simulink library "dspmlti4"  (Simulink 8.2)
settings: Solver=ode45  SolverMode=SingleTasking  StartTime=0.0  StopTime=10.0  RelTol=1e-3
undefined symbols (not defined in the file): Hm_decim, Hm_firdecim, Hm_firinterp, Hm_firsrc, Hm_interp
libraries: simulink x1
settings Model: RequirementInfo=9  Creator=tbryan  LastModifiedBy=jibrahim  CovMetricSettings=d  ExtModeAutoUpdateStatusClock=off

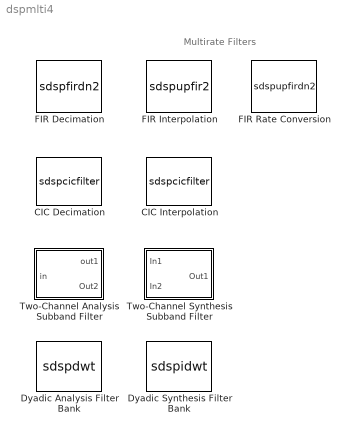
== system dspmlti4 ==
  note: Multirate Filters
  CIC Decimation : S-Function  DialogController=dspdialog.CICDecimation  FunctionName=sdspcicfilter  Parameters=filtFrom,a.ftype,a.R,a.M,a.N,filterInternals,a.section2NWL,a.section2NFL,a.outWL,a.outFL,a.states,framing,1,RateOptions,a.InputWL,a.InputFL  EnableBusSupport=off  mask(CIC Decimation){filtFrom=Dialog, filtobj=Hm_decim, ftype=Decimator, R=2, M=1, N=2, filterInternals=Full precision, BPS=[16 16 16 16], FLPS=0, outputWordLength=32, outputFracLength=0, launchFVT=off, framing=Maintain input frame rate, RateOptions=Enforce single-rate}
      mask prompts: filtFrom "Filter specified via:"; filtobj "Multirate filter variable:"; ftype "Filter structure:"; R "Decimation factor (R):"; M "Differential delay (M):"; N "Number of stages (N):"; filterInternals "Filter internals:"; BPS "Word length for each of the (2*N) filter sections:"; FLPS "Fraction length for each of the (2*N) filter sections:"; outputWordLength "Output word length:"; outputFracLength "Output fraction length:"; launchFVT "Launch Filter Visualization Tool (FVTool)"; RateOptions "Rate options:"
      mask help:
      | Apply a Cascaded Integrator-Comb Decimator filter to the input signal.
      |
      | The inputs and outputs of this block have a signed fixed-point data type with zero bias. You must have a Fixed-Point Designer license to use this block.
      mask init:
      | if filtFrom == 1
      |   str  = dspblkcicfilter('icon',gcbh,filtFrom,'Decimation');
      |   a = dspblkcicfilter('init',gcbh,filtFrom,R,M,N,BPS,FLPS,outputWordLength,outputFracLength,filterInternals);
      | else
      |   str  = dspblkcicfilter('icon',gcbh,filtFrom);
      |   a = dspblkcicfilter('init',gcbh,filtFrom,'Decimation',filtobj);
      | end
      | dspblkcicfilter('initCICDecim',gcbh,filtFrom);
      settings: DeleteFcn=dspLinkFVTool2Mask(gcbh,'close')
      mask Help: eval('blocksethelp');
      mask TypeOptions filtFrom: Dialog | Multirate object in workspace
      mask TypeOptions ftype: Decimator | Zero-latency decimator
      mask TypeOptions filterInternals: Full precision | Minimum section word lengths | Specify word lengths | Binary point scaling
      mask TypeOptions framing: Maintain input frame rate | Maintain input frame size
      mask TypeOptions RateOptions: Enforce single-rate processing | Allow multirate processing | Inherit from input (this choice will be removed - see release notes)
      mask Display: disp(str);
  CIC Interpolation : S-Function  DialogController=dspdialog.CICInterpolation  FunctionName=sdspcicfilter  Parameters=filtFrom,a.ftype,a.R,a.M,a.N,filterInternals,a.section2NWL,a.section2NFL,a.outWL,a.outFL,a.states,framing,InputProcessing,1,a.InputWL, a.InputFL  EnableBusSupport=off  mask(CIC Interpolation){filtFrom=Dialog, filtobj=Hm_interp, ftype=Interpolator, R=2, M=1, N=2, filterInternals=Full precision, BPS=[16 16 16 16], FLPS=0, outputWordLength=32, outputFracLength=0, launchFVT=off, framing=Enforce single-rate, InputProcessing=Columns as channels (frame based)}
      mask prompts: filtFrom "Filter specified via:"; filtobj "Multirate filter variable:"; ftype "Filter structure:"; R "Interpolation factor (R):"; M "Differential delay (M):"; N "Number of stages (N):"; filterInternals "Filter internals:"; BPS "Word length for each of the (2*N) filter stages:"; FLPS "Fraction length for each of the (2*N) filter stages:"; outputWordLength "Output word length:"; outputFracLength "Output fraction length:"; launchFVT "Launch Filter Visualization Tool (FVTool)"; InputProcessing "Input processing:"
      mask help:
      | Apply a Cascaded Integrator-Comb Interpolator filter to the input signal.
      |
      | The inputs and outputs of this block have a signed fixed-point data type with zero bias. You must have a Fixed-Point Designer license to use this block.
      mask init:
      | if filtFrom == 1
      |   str  = dspblkcicfilter('icon',gcbh,filtFrom,'Interpolation');
      |   a = dspblkcicfilter('init',gcbh,filtFrom,R,M,N,BPS,FLPS,outputWordLength,outputFracLength,filterInternals);
      | else
      |   str  = dspblkcicfilter('icon',gcbh,filtFrom);
      |   a = dspblkcicfilter('init',gcbh,filtFrom,'Interpolation',filtobj);
      | end
      | framing = dspblkcicfilter('initCICInterp',gcbh,filtFrom,framing);
      settings: DeleteFcn=dspLinkFVTool2Mask(gcbh,'close')
      mask Help: eval('blocksethelp');
      mask TypeOptions filtFrom: Dialog | Multirate object in workspace
      mask TypeOptions ftype: Interpolator | Zero-latency interpolator
      mask TypeOptions filterInternals: Full precision | Minimum section word lengths | Specify word lengths | Binary point scaling
      mask TypeOptions framing: Enforce single-rate processing | Allow multirate processing | Maintain input frame rate | Maintain input frame size
      mask TypeOptions InputProcessing: Columns as channels (frame based) | Elements as channels (sample based) | Inherited (this choice will be removed - see release notes)
      mask Display: disp(str);
  Dyadic Analysis Filter Bank : S-Function  FunctionName=sdspdwt  Parameters=phl, phh, NumLevels, tree, Output  EnableBusSupport=off  mask(Dyadic Analysis Filter Bank){Wname=User-defined, OrdRec_ordDec=[1 / 1], Order=2, LPF=[0.0352   -0.0854   -0.1350   0.4599   0.8069   0.3327], HPF=[-0.3327    0.8069   -0.4599   -0.1350    0.0854    0.0352], NumLevels=2, tree=Asymmetric, Output=Multiple ports}
      mask prompts: Wname "Filter:"; OrdRec_ordDec "Filter order [synthesis / analysis]:"; Order "Wavelet order:"; LPF "Lowpass FIR filter coefficients:"; HPF "Highpass FIR filter coefficients:"; NumLevels "Number of levels:"; tree "Tree structure:"
      mask help:
      | Compute the Discrete Wavelet Transform or decompose a signal into subbands with smaller bandwidths and slower sample rates. This block uses a filter bank with lowpass and highpass FIR filters that you specify either directly on the block mask, or using wavelets from the Wavelet Toolbox. The lowpass and highpass filters are usually half-band filters designed to complement each other.
      |
      | Inputs are always interpreted as frames. The frame size must be a multiple of 2^n, where you specify n in the 'Number of levels' parameter. When the 'Output' parameter is set to 'Multiple ports', the block outputs each subband from a different port as a vector or matrix. The topmost port outputs the subband with the highest frequency band. When the 'Output' parameter is set to 'Single port', the block outputs one vector or matrix of concatenated subbands.
      mask init:
      | [x,y, str] = dspblkdwt('icon');
      | wname_str = get_param(gcb, 'Wname');
      | OrdRec_ordDec_str = get_param(gcb, 'OrdRec_ordDec');
      | [phl, phh] = dspblkdwt('init', true, LPF, HPF, tree, wname_str, Order, OrdRec_ordDec_str);
      mask Help: eval('blocksethelp');
      mask TypeOptions Wname: User-defined | Haar | Daubechies | Symlets | Coiflets | Biorthogonal | Reverse Biorthogonal | Discrete Meyer
      mask Callback Wname: dspblkdwt
      mask TypeOptions OrdRec_ordDec: [1 / 1] | [1 / 3] | [1 / 5] | [2 / 2] | [2 / 4] | [2 / 6] | [2 / 8] | [3 / 1] | [3 / 3] | [3 / 5] | [3 / 7] | [3 / 9] | [4 / 4] | [5 / 5] | [6 / 8]
      mask TypeOptions tree: Asymmetric | Symmetric
      mask TypeOptions Output: Single port | Multiple ports
      mask Display:
      | plot(x,y)
      | text(0.08,0.1,str)
  Dyadic Synthesis Filter Bank : S-Function  FunctionName=sdspidwt  Parameters=phl, phh, NumLevels, tree, Input  EnableBusSupport=off  mask(Dyadic Synthesis Filter Bank){Wname=User-defined, OrdRec_ordDec=[1 / 1], Order=2, LPF=[0.3327    0.8069    0.4599   -0.1350   -0.0854    0.0352], HPF=[0.0352    0.0854   -0.1350   -0.4599    0.8069   -0.3327], NumLevels=2, tree=Asymmetric, Input=Multiple ports}
      mask prompts: Wname "Filter:"; OrdRec_ordDec "Filter order [synthesis, analysis]:"; Order "Wavelet order:"; LPF "Lowpass FIR filter coefficients:"; HPF "Highpass FIR filter coefficients:"; NumLevels "Number of levels:"; tree "Tree Structure:"
      mask help:
      | Compute the Inverse Discrete Wavelet Transform or reconstruct a signal from subbands with smaller bandwidths and slower sample rates. This block uses a filter bank with lowpass and highpass FIR filters that you specify either directly on the block mask, or using wavelets from the Wavelet Toolbox. The lowpass and highpass filters are usually half-band filters designed to complement each other.
      |
      | When 'Input' is set to 'Multiple ports', you must provide each subband to the block through a different input port as a vector or matrix. You should input the highest frequency band through the topmost port. When 'Input' is set to 'Single port', the block input must be a vector or matrix of concatenated subbands.
      mask init:
      | [x,y,str] = dspblkidwt('icon');
      | wname_str = get_param(gcb, 'Wname');
      | OrdRec_ordDec_str = get_param(gcb, 'OrdRec_ordDec');
      | [phl, phh] = dspblkidwt('init', true, LPF, HPF, tree, wname_str, Order, OrdRec_ordDec_str);
      mask Help: eval('blocksethelp');
      mask TypeOptions Wname: User-defined | Haar | Daubechies | Symlets | Coiflets | Biorthogonal | Reverse Biorthogonal | Discrete Meyer
      mask Callback Wname: dspblkidwt
      mask TypeOptions OrdRec_ordDec: [1 / 1] | [1 / 3] | [1 / 5] | [2 / 2] | [2 / 4] | [2 / 6] | [2 / 8] | [3 / 1] | [3 / 3] | [3 / 5] | [3 / 7] | [3 / 9] | [4 / 4] | [5 / 5] | [6 / 8]
      mask TypeOptions tree: Asymmetric | Symmetric
      mask TypeOptions Input: Single port | Multiple ports
      mask Display:
      | plot(x,y)
      | text(0.08,0.1,str)
  FIR Decimation : S-Function  DialogController=dspdialog.FIRDecimation  DialogControllerArgs=DataTag3  FunctionName=sdspfirdn2  Parameters=a.CoeffSource,a.h,a.D,framing,InputProcessing,inputOffset,a.outBufIC,a.filtStruct,dtInfo.arithmetic,dtInfo.inputWordLength,dtInfo.inputFracLength,firstCoeffMin,firstCoeffMax,outputMin,outputMax,dtInfo.firstCoeffMode,dtInfo.firstCoeffWordLength,dtInfo.firstCoeffFracLength,dtInfo.prodOutputMode,dtInfo.prodOutputWordLength,dtInfo.prodOutputFracLength,dtInfo.accumMode,dtInfo.accumWordLength,dtInfo.accumFracLength,dtInfo.outputMode,dtInfo.outputWordLength,dtInfo.outputFracLength,dtInfo.roundingMode,dtInfo.overflowMode  EnableBusSupport=off  mask(FIR Decimation){h=fir1(35,0.4), D=2, filtStruct=Direct form, framing=Enforce single-rate, inputOffset=0, outputBufInitCond=0, InputProcessing=Columns as channels (frame based), additionalParams=off, allowOverrides=off, firstCoeffMode=Same word length as input, firstCoeffWordLength=16, firstCoeffFracLength=15, firstCoeffDataTypeStr=Inherit: Same word length as input, firstCoeffLastDataTypeStr=Inherit: Same word length as input, firstCoeffMin=[], firstCoeffMax=[], outputMode=Same as accumulator, outputWordLength=16, outputFracLength=15, outputDataTypeStr=Inherit: Same as accumulator, outputLastDataTypeStr=Inherit: Same as accumulator, outputMin=[], outputMax=[], accumMode=Inherit via internal rule, accumWordLength=32, accumFracLength=30, accumDataTypeStr=Inherit: Inherit via internal rule, accumLastDataTypeStr=Inherit: Inherit via internal rule, prodOutputMode=Inherit via internal rule, prodOutputWordLength=32, prodOutputFracLength=30, prodOutputDataTypeStr=Inherit: Inherit via internal rule, prodOutputLastDataTypeStr=Inherit: Inherit via internal rule, roundingMode=Floor, overflowMode=off, LockScale=off, FilterSource=Specify via dialog, FilterObject=Hm_firdecim}
      mask prompts: h "FIR filter coefficients:"; D "Decimation factor:"; filtStruct "Filter structure:"; inputOffset "Input offset:"; outputBufInitCond "Output buffer initial conditions:"; InputProcessing "Input processing:"; additionalParams "--------------- Show additional parameters ---------------"; allowOverrides "Allow overrides from DSP Fixed-Point Attributes blocks"; firstCoeffMode "Fixed-point coefficient attributes:"; firstCoeffWordLength "Coefficient word length:"; firstCoeffFracLength "Coefficient fraction length:"; firstCoeffDataTypeStr "Coefficients data type string:"; firstCoeffLastDataTypeStr "Last coefficients data type string:"; firstCoeffMin "Coefficients minimum:"; firstCoeffMax "Coefficients maximum:"; outputMode "Fixed-point output attributes:"; outputWordLength "Output word length:"; outputFracLength "Output fractional length:"; outputDataTypeStr "Output data type string:"; outputLastDataTypeStr "Last output data type string:"; outputMin "Output minimum:"; outputMax "Output maximum:"; accumMode "Fixed-point accumulator attributes:"; accumWordLength "Accumulator word length:"; accumFracLength "Accumulator fraction length:"; accumDataTypeStr "Accum data type string:"; accumLastDataTypeStr "Last accum data type string:"; prodOutputMode "Fixed-point product output attributes:"; prodOutputWordLength "Product output word length:"; prodOutputFracLength "Product output fraction length:"; prodOutputDataTypeStr "ProdOutput data type string:"; prodOutputLastDataTypeStr "Last prodOutput data type string:"; roundingMode "Round integer calculations towards:"; overflowMode "Saturate on integer overflow"; LockScale "Lock scaling"; FilterSource "Coefficient source:"; FilterObject "Filter object:"
      mask help: Apply an FIR filter to the input signal, then downsample the signal by an integer-valued factor. The block implements the FIR filter using a polyphase filter structure.
      mask init:
      | dtRows = dspblkGetFIRMultirateFiltersDTRowInfo();
      | if FilterSource == 1
      |     str = dspblkfirdn2(gcbh,'icon',FilterSource,D);
      |     [a,dtInfo,framing] = dspblkfirdn2(gcbh,'setup',FilterSource,dtRows,h,D,filtStruct,outputBufInitCond,framing);
      | else
      |     str = dspblkfirdn2(gcbh,'icon',FilterSource,FilterObject);
      |     [a,dtInfo,framing] = dspblkfirdn2(gcbh,'setup',FilterSource,FilterObject,framing);
      | end
      | dspblkfirdn2(gcbh,'init',FilterSource);
      settings: DeleteFcn=dspLinkFVTool2Mask(gcbh,'close')
      mask Help: eval('blocksethelp');
      mask TypeOptions filtStruct: Direct form | Direct form transposed
      mask TypeOptions framing: Enforce single-rate processing | Allow multirate processing | Maintain input frame size | Maintain input frame rate
      mask TypeOptions InputProcessing: Columns as channels (frame based) | Elements as channels (sample based) | Inherited (this choice will be removed - see release notes)
      mask TypeOptions firstCoeffMode: Same word length as input | Specify word length | Binary point scaling | Slope and bias scaling | User-defined
      mask TypeOptions outputMode: Same as accumulator | Same as product output | Same as input | Binary point scaling | Slope and bias scaling | User-defined
      mask TypeOptions accumMode: Inherit via internal rule | Same as product output | Same as input | Binary point scaling | Slope and bias scaling | User-defined
      mask TypeOptions prodOutputMode: Inherit via internal rule | Same as input | Binary point scaling | Slope and bias scaling | User-defined
      mask TypeOptions roundingMode: Ceiling | Convergent | Floor | Nearest | Round | Simplest | Zero
      mask TypeOptions FilterSource: Specify via dialog | Filter object
      mask Display: disp(str)
  FIR Interpolation : S-Function  DialogController=dspdialog.FIRInterpolation  DialogControllerArgs=DataTag5  FunctionName=sdspupfir2  Parameters=a.CoeffSource,a.h,a.L,framing,InputProcessing,a.outBufIC,dtInfo.arithmetic,dtInfo.inputWordLength,dtInfo.inputFracLength,firstCoeffMin,firstCoeffMax,outputMin,outputMax,dtInfo.firstCoeffMode,dtInfo.firstCoeffWordLength,dtInfo.firstCoeffFracLength,dtInfo.prodOutputMode,dtInfo.prodOutputWordLength,dtInfo.prodOutputFracLength,dtInfo.accumMode,dtInfo.accumWordLength,dtInfo.accumFracLength,dtInfo.outputMode,dtInfo.outputWordLength,dtInfo.outputFracLength,dtInfo.roundingMode,dtInfo.overflowMode  EnableBusSupport=off  mask(FIR Interpolation){h=fir1(15,1/4), L=3, framing=Enforce single-rate processing, outputBufInitCond=0, InputProcessing=Columns as channels (frame based), additionalParams=off, allowOverrides=on, firstCoeffMode=Same word length as input, firstCoeffWordLength=16, firstCoeffFracLength=15, firstCoeffDataTypeStr=Inherit: Same word length as input, firstCoeffLastDataTypeStr=Inherit: Same word length as input, firstCoeffMin=[], firstCoeffMax=[], outputMode=Same as accumulator, outputWordLength=16, outputFracLength=15, outputDataTypeStr=Inherit: Same as accumulator, outputLastDataTypeStr=Inherit: Same as accumulator, outputMin=[], outputMax=[], accumMode=Inherit via internal rule, accumWordLength=32, accumFracLength=30, accumDataTypeStr=Inherit: Inherit via internal rule, accumLastDataTypeStr=Inherit: Inherit via internal rule, prodOutputMode=Inherit via internal rule, prodOutputWordLength=32, prodOutputFracLength=30, prodOutputDataTypeStr=Inherit: Inherit via internal rule, prodOutputLastDataTypeStr=Inherit: Inherit via internal rule, roundingMode=Floor, overflowMode=off, LockScale=off, FilterSource=Specify via dialog, FilterObject=Hm_firinterp}
      mask prompts: h "FIR filter coefficients:"; L "Interpolation factor:"; outputBufInitCond "Output buffer initial conditions:"; InputProcessing "Input processing:"; additionalParams "--------------- Show additional parameters ---------------"; allowOverrides "Allow overrides from DSP Fixed-Point Attributes blocks"; firstCoeffMode "Fixed-point coefficient attributes:"; firstCoeffWordLength "Coefficient word length:"; firstCoeffFracLength "Coefficient fraction length:"; firstCoeffDataTypeStr "Coefficients data type string:"; firstCoeffLastDataTypeStr "Last coefficients data type string:"; firstCoeffMin "Coefficients minimum:"; firstCoeffMax "Coefficients maximum:"; outputMode "Fixed-point output attributes:"; outputWordLength "Output word length:"; outputFracLength "Output fractional length:"; outputDataTypeStr "Output data type string:"; outputLastDataTypeStr "Last output data type string:"; outputMin "Output minimum:"; outputMax "Output maximum:"; accumMode "Fixed-point accumulator attributes:"; accumWordLength "Accumulator word length:"; accumFracLength "Accumulator fraction length:"; accumDataTypeStr "Accum data type string:"; accumLastDataTypeStr "Last accum data type string:"; prodOutputMode "Fixed-point product output attributes:"; prodOutputWordLength "Product output word length:"; prodOutputFracLength "Product output fraction length:"; prodOutputDataTypeStr "ProdOutput data type string:"; prodOutputLastDataTypeStr "Last prodOutput data type string:"; roundingMode "Round integer calculations towards:"; overflowMode "Saturate on integer overflow"; LockScale "Lock scaling"; FilterSource "Coefficient source:"; FilterObject "Filter object:"
      mask help: Upsample the input signal by an integer-valued factor, then apply an FIR filter. The block scales the filter coefficients by the interpolation factor and implements the FIR filter using a polyphase structure.
      mask init:
      | dtRows = dspblkGetFIRMultirateFiltersDTRowInfo();
      | if FilterSource == 1
      |     str = dspblkupfir2(gcbh,'icon',FilterSource,L);
      |     [a,dtInfo,framing] = dspblkupfir2(gcbh,'setup',FilterSource,dtRows,h,L,outputBufInitCond,framing);
      | else
      |     str = dspblkupfir2(gcbh,'icon',FilterSource,FilterObject);
      |     [a,dtInfo,framing] = dspblkupfir2(gcbh,'setup',FilterSource,FilterObject,framing);
      | end
      | dspblkupfir2(gcbh,'init',FilterSource);
      settings: DeleteFcn=dspLinkFVTool2Mask(gcbh,'close')
      mask Help: eval('blocksethelp');
      mask TypeOptions framing: Enforce single-rate processing | Allow multirate processing | Maintain input frame size | Maintain input frame rate
      mask TypeOptions InputProcessing: Columns as channels (frame based) | Elements as channels (sample based) | Inherited (this choice will be removed - see release notes)
      mask TypeOptions firstCoeffMode: Same word length as input | Specify word length | Binary point scaling | Slope and bias scaling | User-defined
      mask TypeOptions outputMode: Same as accumulator | Same as product output | Same as input | Binary point scaling | Slope and bias scaling | User-defined
      mask TypeOptions accumMode: Inherit via internal rule | Same as product output | Same as input | Binary point scaling | Slope and bias scaling | User-defined
      mask TypeOptions prodOutputMode: Inherit via internal rule | Same as input | Binary point scaling | Slope and bias scaling | User-defined
      mask TypeOptions roundingMode: Ceiling | Convergent | Floor | Nearest | Round | Simplest | Zero
      mask TypeOptions FilterSource: Specify via dialog | Filter object
      mask Display: disp(str)
  FIR Rate Conversion : S-Function  DialogController=dspdialog.FIRSampleRateConversion  DialogControllerArgs=DataTag6  FunctionName=sdspupfirdn2  Parameters=a.CoeffSource,a.h,a.L,a.M,dtInfo.arithmetic,dtInfo.inputWordLength,dtInfo.inputFracLength,firstCoeffMin,firstCoeffMax,outputMin,outputMax,dtInfo.firstCoeffMode,dtInfo.firstCoeffWordLength,dtInfo.firstCoeffFracLength,dtInfo.prodOutputMode,dtInfo.prodOutputWordLength,dtInfo.prodOutputFracLength,dtInfo.accumMode,dtInfo.accumWordLength,dtInfo.accumFracLength,dtInfo.outputMode,dtInfo.outputWordLength,dtInfo.outputFracLength,dtInfo.roundingMode,dtInfo.overflowMode  EnableBusSupport=off  mask(FIR Rate Conversion){L=3, h=firpm(70,[0 .28 .32 1],[1 1 0 0]), M=2, additionalParams=off, allowOverrides=on, firstCoeffMode=Same word length as input, firstCoeffWordLength=16, firstCoeffFracLength=15, firstCoeffDataTypeStr=Inherit: Same word length as input, firstCoeffLastDataTypeStr=Inherit: Same word length as input, firstCoeffMin=[], firstCoeffMax=[], outputMode=Same as accumulator, outputWordLength=16, outputFracLength=15, outputDataTypeStr=Inherit: Same as accumulator, outputLastDataTypeStr=Inherit: Same as accumulator, outputMin=[], outputMax=[], accumMode=Inherit via internal rule, accumWordLength=32, accumFracLength=30, accumDataTypeStr=Inherit: Inherit via internal rule, accumLastDataTypeStr=Inherit: Inherit via internal rule, prodOutputMode=Inherit via internal rule, prodOutputWordLength=32, prodOutputFracLength=30, prodOutputDataTypeStr=Inherit: Inherit via internal rule, prodOutputLastDataTypeStr=Inherit: Inherit via internal rule, roundingMode=Floor, overflowMode=off, LockScale=off, FilterSource=Specify via dialog, FilterObject=Hm_firsrc}
      mask prompts: L "Interpolation factor:"; h "FIR filter coefficients:"; M "Decimation factor:"; additionalParams "--------------- Show additional parameters ---------------"; allowOverrides "Allow overrides from DSP Fixed-Point Attributes blocks"; firstCoeffMode "Fixed-point coefficient attributes:"; firstCoeffWordLength "Coefficient word length:"; firstCoeffFracLength "Coefficient fraction length:"; firstCoeffDataTypeStr "Coefficients data type string:"; firstCoeffLastDataTypeStr "Last coefficients data type string:"; firstCoeffMin "Coefficients minimum:"; firstCoeffMax "Coefficients maximum:"; outputMode "Fixed-point output attributes:"; outputWordLength "Output word length:"; outputFracLength "Output fractional length:"; outputDataTypeStr "Output data type string:"; outputLastDataTypeStr "Last output data type string:"; outputMin "Output minimum:"; outputMax "Output maximum:"; accumMode "Fixed-point accumulator attributes:"; accumWordLength "Accumulator word length:"; accumFracLength "Accumulator fraction length:"; accumDataTypeStr "Accum data type string:"; accumLastDataTypeStr "Last accum data type string:"; prodOutputMode "Fixed-point product output attributes:"; prodOutputWordLength "Product output word length:"; prodOutputFracLength "Product output fraction length:"; prodOutputDataTypeStr "ProdOutput data type string:"; prodOutputLastDataTypeStr "Last prodOutput data type string:"; roundingMode "Round integer calculations towards:"; overflowMode "Saturate on integer overflow"; LockScale "Lock scaling"; FilterSource "Coefficient source:"; FilterObject "Filter object:"
      mask help: Upsample the input signal by an integer-valued factor, apply an FIR filter, and downsample the input signal by another integer-valued factor. The block implements the FIR filter using a polyphase structure.
      mask init:
      | blkh   = gcbh;
      | dtRows = dspblkGetFIRMultirateFiltersDTRowInfo();
      | if FilterSource == 1
      |     str = dspblkupfirdn2('icon',FilterSource,L,M);
      |     [a,dtInfo] = dspblkupfirdn2('setup',FilterSource,dtRows,h,L,M);
      | else
      |     str = dspblkupfirdn2('icon',FilterSource,FilterObject);
      |     [a,dtInfo] = dspblkupfirdn2('setup',FilterSource,FilterObject);
      | end
      settings: DeleteFcn=dspLinkFVTool2Mask(gcbh,'close')
      mask Help: eval('blocksethelp');
      mask TypeOptions firstCoeffMode: Same word length as input | Specify word length | Binary point scaling | Slope and bias scaling | User-defined
      mask TypeOptions outputMode: Same as accumulator | Same as product output | Same as input | Binary point scaling | Slope and bias scaling | User-defined
      mask TypeOptions accumMode: Inherit via internal rule | Same as product output | Same as input | Binary point scaling | Slope and bias scaling | User-defined
      mask TypeOptions prodOutputMode: Inherit via internal rule | Same as input | Binary point scaling | Slope and bias scaling | User-defined
      mask TypeOptions roundingMode: Ceiling | Convergent | Floor | Nearest | Round | Simplest | Zero
      mask TypeOptions FilterSource: Specify via dialog | Filter object
      mask Display: disp(str)
  Two-Channel Analysis Subband Filter : Subsystem  DialogController=dspDDGCreate  DialogControllerArgs=DataTag8  mask(Two-Channel Analysis Subband Filter){lpf=[0.0352   -0.0854   -0.1350   0.4599   0.8069   0.3327], hpf=[-0.3327    0.8069   -0.4599   -0.1350    0.0854    0.0352], framing=Enforce single-rate processing, InputProcessing=Columns as channels (frame based), additionalParams=off, allowOverrides=off, firstCoeffMode=Same word length as input, firstCoeffWordLength=16, firstCoeffFracLength=15, firstCoeffDataTypeStr=Inherit: Same word length as input, firstCoeffLastDataTypeStr=Inherit: Same word length as input, firstCoeffMin=[], firstCoeffMax=[], outputMode=Same as accumulator, outputWordLength=16, outputFracLength=14, outputDataTypeStr=Inherit: Same as accumulator, outputLastDataTypeStr=Inherit: Same as accumulator, outputMin=[], outputMax=[], accumMode=Inherit via internal rule, accumWordLength=32, accumFracLength=30, accumDataTypeStr=Inherit: Inherit via internal rule, accumLastDataTypeStr=Inherit: Inherit via internal rule, prodOutputMode=Inherit via internal rule, prodOutputWordLength=32, prodOutputFracLength=30, prodOutputDataTypeStr=Inherit: Inherit via internal rule, prodOutputLastDataTypeStr=Inherit: Inherit via internal rule, roundingMode=Floor, overflowMode=off, LockScale=off}
      mask prompts: lpf "Lowpass FIR filter coefficients:"; hpf "Highpass FIR filter coefficients:"; InputProcessing "Input processing:"; additionalParams "--------------- Show additional parameters ---------------"; allowOverrides "Allow overrides from DSP Fixed-Point Attributes blocks"; firstCoeffMode "Fixed-point coefficient attributes:"; firstCoeffWordLength "Coefficient word length:"; firstCoeffFracLength "Coefficient fraction length:"; firstCoeffDataTypeStr "Coefficients data type string:"; firstCoeffLastDataTypeStr "Last coefficients data type string:"; firstCoeffMin "Coefficients minimum:"; firstCoeffMax "Coefficients maximum:"; outputMode "Fixed-point output attributes:"; outputWordLength "Output word length:"; outputFracLength "Output fraction length:"; outputDataTypeStr "Output data type string:"; outputLastDataTypeStr "Last output data type string:"; outputMin "Output minimum:"; outputMax "Output maximum:"; accumMode "Fixed-point accumulator attributes:"; accumWordLength "Accumulator word length:"; accumFracLength "Accumulator fraction length:"; accumDataTypeStr "Accum data type string:"; accumLastDataTypeStr "Last accum data type string:"; prodOutputMode "Fixed-point product output attributes:"; prodOutputWordLength "Product output word length:"; prodOutputFracLength "Product output fraction length:"; prodOutputDataTypeStr "ProdOutput data type string:"; prodOutputLastDataTypeStr "Last prodOutput data type string:"; roundingMode "Round integer calculations towards:"; overflowMode "Saturate on integer overflow"; LockScale "Lock scaling"
      mask help: Decompose a signal into a high-frequency subband (Hi band) and a low-frequency subband (Lo band) using the specified highpass and lowpass FIR filters. Each subband has half the bandwidth and half the sample rate of the original signal. Usually, the highpass and lowpass filters should be half-band filters designed to complement each other.
      mask init:
      | blkh   = gcbh;
      | dtRows = dspblkGetFIRMultirateFiltersDTRowInfo();
      | dtInfo = dspGetUDTFixptDataTypeInfo(blkh, dtRows, true); 
      | [hpf,lpf,framing] = dspblk2chabank2(blkh,hpf,lpf,framing);
      mask Help: eval('blocksethelp');
      mask TypeOptions framing: Enforce single-rate processing | Allow multirate processing | Maintain input frame size | Maintain input frame rate
      mask TypeOptions InputProcessing: Columns as channels (frame based) | Elements as channels (sample based) | Inherited (this choice will be removed - see release notes)
      mask TypeOptions firstCoeffMode: Same word length as input | Specify word length | Binary point scaling | Slope and bias scaling | User-defined
      mask TypeOptions outputMode: Same as accumulator | Same as product output | Same as input | Binary point scaling | Slope and bias scaling | User-defined
      mask TypeOptions accumMode: Inherit via internal rule | Same as product output | Same as input | Binary point scaling | Slope and bias scaling | User-defined
      mask TypeOptions prodOutputMode: Inherit via internal rule | Same as input | Binary point scaling | Slope and bias scaling | User-defined
      mask TypeOptions roundingMode: Ceiling | Convergent | Floor | Nearest | Round | Simplest | Zero
      mask Display:
      | disp('');
      | port_label('output', 1, 'Hi band');
      | port_label('output', 2, 'Lo band');
  Two-Channel Synthesis Subband Filter : Subsystem  DialogController=dspDDGCreate  DialogControllerArgs=DataTag10  mask(Two-Channel Synthesis Subband Filter){lpf=[0.3327    0.8069    0.4599   -0.1350   -0.0854    0.0352], hpf=[0.0352    0.0854   -0.1350   -0.4599    0.8069   -0.3327], framing=Enforce single-rate processing, InputProcessing=Columns as channels (frame based), additionalParams=off, allowOverrides=off, firstCoeffMode=Same word length as input, firstCoeffWordLength=16, firstCoeffFracLength=15, firstCoeffDataTypeStr=Inherit: Same word length as input, firstCoeffLastDataTypeStr=Inherit: Same word length as input, firstCoeffMin=[], firstCoeffMax=[], outputMode=Same as accumulator, outputWordLength=16, outputFracLength=14, outputDataTypeStr=Inherit: Same as accumulator, outputLastDataTypeStr=Inherit: Same as accumulator, outputMin=[], outputMax=[], accumMode=Inherit via internal rule, accumWordLength=32, accumFracLength=30, accumDataTypeStr=Inherit: Inherit via internal rule, accumLastDataTypeStr=Inherit: Inherit via internal rule, prodOutputMode=Inherit via internal rule, prodOutputWordLength=32, prodOutputFracLength=30, prodOutputDataTypeStr=Inherit: Inherit via internal rule, prodOutputLastDataTypeStr=Inherit: Inherit via internal rule, roundingMode=Floor, overflowMode=off, LockScale=off}
      mask prompts: lpf "Lowpass FIR filter coefficients:"; hpf "Highpass FIR filter coefficients:"; InputProcessing "Input processing:"; additionalParams "--------------- Show additional parameters ---------------"; allowOverrides "Allow overrides from DSP Fixed-Point Attributes blocks"; firstCoeffMode "Fixed-point coefficient attributes:"; firstCoeffWordLength "Coefficient word length:"; firstCoeffFracLength "Coefficient fraction length:"; firstCoeffDataTypeStr "Coefficients data type string:"; firstCoeffLastDataTypeStr "Last coefficients data type string:"; firstCoeffMin "Coefficients minimum:"; firstCoeffMax "Coefficients maximum:"; outputMode "Fixed-point output attributes:"; outputWordLength "Output word length:"; outputFracLength "Output fraction length:"; outputDataTypeStr "Output data type string:"; outputLastDataTypeStr "Last output data type string:"; outputMin "Output minimum:"; outputMax "Output maximum:"; accumMode "Fixed-point accumulator attributes:"; accumWordLength "Accumulator word length:"; accumFracLength "Accumulator fraction length:"; accumDataTypeStr "Accum data type string:"; accumLastDataTypeStr "Last accum data type string:"; prodOutputMode "Fixed-point product output attributes:"; prodOutputWordLength "Product output word length:"; prodOutputFracLength "Product output fraction length:"; prodOutputDataTypeStr "ProdOutput data type string:"; prodOutputLastDataTypeStr "Last prodOutput data type string:"; roundingMode "Round integer calculations towards:"; overflowMode "Saturate on integer overflow"; LockScale "Lock scaling"
      mask help: Reconstruct a signal from a high-frequency subband (Hi band) and a low-frequnecy subband (Lo band) using the specified highpass and lowpass FIR filters. The input subbands should have the same bandwidths and sample rates. Usually, the highpass and lowpass filters should be half-band filters designed to complement each other.
      mask init:
      | blkh   = gcbh;
      | dtRows = dspblkGetFIRMultirateFiltersDTRowInfo();
      | dtInfo = dspGetUDTFixptDataTypeInfo(blkh, dtRows, true);
      | [hpf,lpf,framing] = dspblk2chsbank(blkh,hpf,lpf,framing, ...
      |     dtInfo.roundingMode,dtInfo.overflowMode);
      mask Help: eval('blocksethelp');
      mask TypeOptions framing: Enforce single-rate processing | Allow multirate processing | Maintain input frame size | Maintain input frame rate
      mask TypeOptions InputProcessing: Columns as channels (frame based) | Elements as channels (sample based) | Inherited (this choice will be removed - see release notes)
      mask TypeOptions firstCoeffMode: Same word length as input | Specify word length | Binary point scaling | Slope and bias scaling | User-defined
      mask TypeOptions outputMode: Same as accumulator | Same as product output | Same as input | Binary point scaling | Slope and bias scaling | User-defined
      mask TypeOptions accumMode: Inherit via internal rule | Same as product output | Same as input | Binary point scaling | Slope and bias scaling | User-defined
      mask TypeOptions prodOutputMode: Inherit via internal rule | Same as input | Binary point scaling | Slope and bias scaling | User-defined
      mask TypeOptions roundingMode: Ceiling | Convergent | Floor | Nearest | Round | Simplest | Zero
      mask Display:
      | disp('');
      | port_label('input', 1, 'Hi band');
      | port_label('input', 2, 'Lo band');

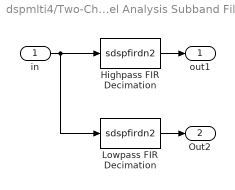
== system dspmlti4/Two-Channel Analysis Subband Filter ==
  in : Inport
  Highpass FIR Decimation : S-Function  FunctionName=sdspfirdn2  Parameters=1,hpf,2,framing,InputProcessing,0,0,1,0,16,15,firstCoeffMin,firstCoeffMax,outputMin,outputMax,dtInfo.firstCoeffMode,dtInfo.firstCoeffWordLength,dtInfo.firstCoeffFracLength,dtInfo.prodOutputMode,dtInfo.prodOutputWordLength,dtInfo.prodOutputFracLength,dtInfo.accumMode,dtInfo.accumWordLength,dtInfo.accumFracLength,dtInfo.outputMode,dtInfo.outputWordLength,dtInfo.outputFracLength,dtInfo.roundingMode,dtInfo.overflowMode  EnableBusSupport=off
  Lowpass FIR Decimation : S-Function  FunctionName=sdspfirdn2  Parameters=1,lpf,2,framing,InputProcessing,0,0,1,0,16,15,firstCoeffMin,firstCoeffMax,outputMin,outputMax,dtInfo.firstCoeffMode,dtInfo.firstCoeffWordLength,dtInfo.firstCoeffFracLength,dtInfo.prodOutputMode,dtInfo.prodOutputWordLength,dtInfo.prodOutputFracLength,dtInfo.accumMode,dtInfo.accumWordLength,dtInfo.accumFracLength,dtInfo.outputMode,dtInfo.outputWordLength,dtInfo.outputFracLength,dtInfo.roundingMode,dtInfo.overflowMode  EnableBusSupport=off
  out1 : Outport
  Out2 : Outport  Port=2
  wires:
  Highpass FIR Decimation/1 -> out1/1
  in/1 -> Lowpass FIR Decimation/1, Highpass FIR Decimation/1
  Lowpass FIR Decimation/1 -> Out2/1

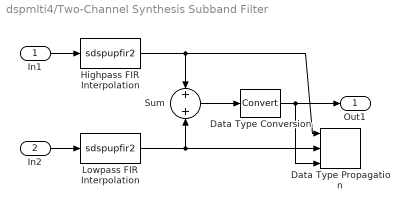
== system dspmlti4/Two-Channel Synthesis Subband Filter ==
  In1 : Inport
  In2 : Inport  Port=2
  Data Type Conversion : DataTypeConversion
  Data Type Propagation : simulink/Signal Attributes/Data Type Propagation  PropDataType=sfix(16)  IfRefDouble=double  IfRefSingle=single  IsSigned=IsSigned1 or IsSigned2  NumBitsBase=NumBits1  NumBitsMult=1  NumBitsAdd=0  NumBitsAllowFinal=1:128  PropScaling=2^-10  ValuesUsedBestPrec=[5 -7]  SlopeBase=Slope1  SlopeMult=1  SlopeAdd=0  BiasBase=Bias1  BiasMult=1  BiasAdd=0
  Highpass FIR Interpolation : S-Function  FunctionName=sdspupfir2  Parameters=1,hpf,2,framing,InputProcessing,0,0,16,15,firstCoeffMin,firstCoeffMax,outputMin,outputMax,dtInfo.firstCoeffMode,dtInfo.firstCoeffWordLength,dtInfo.firstCoeffFracLength,dtInfo.prodOutputMode,dtInfo.prodOutputWordLength,dtInfo.prodOutputFracLength,dtInfo.accumMode,dtInfo.accumWordLength,dtInfo.accumFracLength,dtInfo.outputMode,dtInfo.outputWordLength,dtInfo.outputFracLength,dtInfo.roundingMode,dtInfo.overflowMode  EnableBusSupport=off
  Lowpass FIR Interpolation : S-Function  FunctionName=sdspupfir2  Parameters=1,lpf,2,framing,InputProcessing,0,0,16,15,firstCoeffMin,firstCoeffMax,outputMin,outputMax,dtInfo.firstCoeffMode,dtInfo.firstCoeffWordLength,dtInfo.firstCoeffFracLength,dtInfo.prodOutputMode,dtInfo.prodOutputWordLength,dtInfo.prodOutputFracLength,dtInfo.accumMode,dtInfo.accumWordLength,dtInfo.accumFracLength,dtInfo.outputMode,dtInfo.outputWordLength,dtInfo.outputFracLength,dtInfo.roundingMode,dtInfo.overflowMode  EnableBusSupport=off
  Sum : Sum  Inputs=+|+  InputSameDT=on
  Out1 : Outport
  wires:
  In2/1 -> Lowpass FIR Interpolation/1
  Sum/1 -> Data Type Conversion/1
  In1/1 -> Highpass FIR Interpolation/1
  Lowpass FIR Interpolation/1 -> Data Type Propagation/2, Sum/2
  Highpass FIR Interpolation/1 -> Data Type Propagation/1, Sum/1
  Data Type Conversion/1 -> Out1/1, Data Type Propagation/3
